simulink model "Reciever"  (R2016b)
settings: Solver=VariableStepAuto  StartTime=0.0  StopTime=inf  RelTol=1e-3
libraries: commsdrhw_v2 x1
settings Model: Creator=root  LastModifiedBy=root

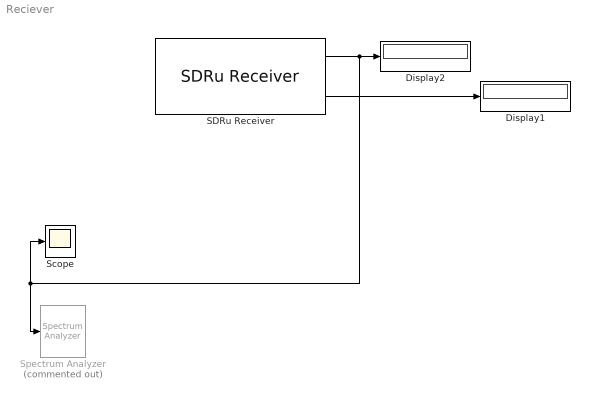
== system Reciever ==
  Display1 : Display
  Display2 : Display
  SDRu Receiver : commsdrhw_v2/SDRu Receiver  SourceLibraryInfo="This block requires <a href=\"http://www.mathworks.com/hardware-support/usrp.html\">Communications System Toolbox Support Package for USRP Radio</a>"  rxtx=rx  platform=N200/N210/USRP2  USRP2_IP='192.168.10.3'  USRP_IP_X300='192.168.10.2'  USRP_IP_X310='192.168.10.2'  USRP_serialNumB200=''  USRP_serialNumB210=''  ChannelMapping=1  centerFrequency=1.57542e9  centerFrequencySrc=Dialog  loOffset=4000  loOffsetSrc=Dialog  PPSSource=Internal  clockSource=Internal  masterClkRateB200=32e6  masterClkRateB210=32e6  masterClkRateX300=200e6  masterClkRateX310=200e6  masterClkRateParam=100e6  gain=71  gainSrc=Dialog  decimInterpSrc=Dialog  decimInterp=512  TransportDataType=int16  USRP2_IP_NUM=[49 57 50 46 49 54 56 46 49 48 46 51]  frameLength=1  outputDatatype=Same as transport data type  overrunUnderrunPort=off  sampleTime=1/(2e6)  HOST_DATA_PORT=0  HOST_CONTROL_PORT=0  USRP2_DATA_PORT=0  USRP2_CONTROL_PORT=0  bufferMode=Continuous streaming  EnableBurstMode=off  NumFramesInBurst=100  USRP_ID='192.168.10.3'
  Scope : Scope
  Spectrum Analyzer : SpectrumAnalyzer  Commented=on
  wires:
  SDRu Receiver/2 -> Display1/1
  SDRu Receiver/1 -> Spectrum Analyzer/1, Scope/1, Display2/1
